simulink model "PV_solarpannel"  (R2019b)
settings: Solver=ode45  StartTime=0.0  StopTime=10.0  RelTol=1e-3  EnableMultiTasking=on
libraries: ee_lib x243, fl_lib x39, nesl_utility x11
(part 2 of 4)

== system PV_solarpannel/Subsystem1/Subsystem9/Subsystem4 ==
  Solar Cell : ee_lib/Sources/Solar Cell  prm=1  Isc=6 A  Voc=0.6 V  Is=1e-6 A  Is2=0 A  Iph=7.34 A  Ir0=1000 W/m^2  ec=1.5  N2=2  Rs=0 Ohm  Rp=Inf Ohm  N_series=1  TIPH1=0 1/K  EG=1.11 eV  TXIS1=3  TXIS2=3  TRS1=0  TRP1=0  Tmeas=25 C  TFIXED=25 C  thermal_mass=100 J/K  initial_temperature=25 degC
      settings: SourceProductName=Simscape Electrical  SourceProductBaseCode=PS
  Solar Cell1 : ee_lib/Sources/Solar Cell  prm=1  Isc=6 A  Voc=0.6 V  Is=1e-6 A  Is2=0 A  Iph=7.34 A  Ir0=1000 W/m^2  ec=1.5  N2=2  Rs=0 Ohm  Rp=Inf Ohm  N_series=1  TIPH1=0 1/K  EG=1.11 eV  TXIS1=3  TXIS2=3  TRS1=0  TRP1=0  Tmeas=25 C  TFIXED=25 C  thermal_mass=100 J/K  initial_temperature=25 degC
      settings: SourceProductName=Simscape Electrical  SourceProductBaseCode=PS
  Solar Cell2 : ee_lib/Sources/Solar Cell  prm=1  Isc=6 A  Voc=0.6 V  Is=1e-6 A  Is2=0 A  Iph=7.34 A  Ir0=1000 W/m^2  ec=1.5  N2=2  Rs=0 Ohm  Rp=Inf Ohm  N_series=1  TIPH1=0 1/K  EG=1.11 eV  TXIS1=3  TXIS2=3  TRS1=0  TRP1=0  Tmeas=25 C  TFIXED=25 C  thermal_mass=100 J/K  initial_temperature=25 degC
      settings: SourceProductName=Simscape Electrical  SourceProductBaseCode=PS
  Conn1 : PMIOPort  Side=Left
  Conn2 : PMIOPort  Port=2  Side=Right
  Conn3 : PMIOPort  Port=3  Side=Left
  connections:
  Solar Cell/LConn2 -- Conn2/RConn1
  Solar Cell/LConn1 -- Conn1/RConn1 -- Solar Cell2/LConn1 -- Solar Cell1/LConn1
  Solar Cell1/RConn1 -- Solar Cell2/LConn2
  Solar Cell/RConn1 -- Solar Cell1/LConn2
  Solar Cell2/RConn1 -- Conn3/RConn1

== system PV_solarpannel/Subsystem1/Subsystem9/Subsystem5 ==
  Solar Cell : ee_lib/Sources/Solar Cell  prm=1  Isc=6 A  Voc=0.6 V  Is=1e-6 A  Is2=0 A  Iph=7.34 A  Ir0=1000 W/m^2  ec=1.5  N2=2  Rs=0 Ohm  Rp=Inf Ohm  N_series=1  TIPH1=0 1/K  EG=1.11 eV  TXIS1=3  TXIS2=3  TRS1=0  TRP1=0  Tmeas=25 C  TFIXED=25 C  thermal_mass=100 J/K  initial_temperature=25 degC
      settings: SourceProductName=Simscape Electrical  SourceProductBaseCode=PS
  Solar Cell1 : ee_lib/Sources/Solar Cell  prm=1  Isc=6 A  Voc=0.6 V  Is=1e-6 A  Is2=0 A  Iph=7.34 A  Ir0=1000 W/m^2  ec=1.5  N2=2  Rs=0 Ohm  Rp=Inf Ohm  N_series=1  TIPH1=0 1/K  EG=1.11 eV  TXIS1=3  TXIS2=3  TRS1=0  TRP1=0  Tmeas=25 C  TFIXED=25 C  thermal_mass=100 J/K  initial_temperature=25 degC
      settings: SourceProductName=Simscape Electrical  SourceProductBaseCode=PS
  Solar Cell2 : ee_lib/Sources/Solar Cell  prm=1  Isc=6 A  Voc=0.6 V  Is=1e-6 A  Is2=0 A  Iph=7.34 A  Ir0=1000 W/m^2  ec=1.5  N2=2  Rs=0 Ohm  Rp=Inf Ohm  N_series=1  TIPH1=0 1/K  EG=1.11 eV  TXIS1=3  TXIS2=3  TRS1=0  TRP1=0  Tmeas=25 C  TFIXED=25 C  thermal_mass=100 J/K  initial_temperature=25 degC
      settings: SourceProductName=Simscape Electrical  SourceProductBaseCode=PS
  Conn1 : PMIOPort  Side=Left
  Conn2 : PMIOPort  Port=2  Side=Right
  Conn3 : PMIOPort  Port=3  Side=Left
  connections:
  Solar Cell/LConn2 -- Conn2/RConn1
  Solar Cell/LConn1 -- Conn1/RConn1 -- Solar Cell2/LConn1 -- Solar Cell1/LConn1
  Solar Cell1/RConn1 -- Solar Cell2/LConn2
  Solar Cell/RConn1 -- Solar Cell1/LConn2
  Solar Cell2/RConn1 -- Conn3/RConn1

== system PV_solarpannel/Subsystem1/Subsystem9/Subsystem6 ==
  Solar Cell : ee_lib/Sources/Solar Cell  prm=1  Isc=6 A  Voc=0.6 V  Is=1e-6 A  Is2=0 A  Iph=7.34 A  Ir0=1000 W/m^2  ec=1.5  N2=2  Rs=0 Ohm  Rp=Inf Ohm  N_series=1  TIPH1=0 1/K  EG=1.11 eV  TXIS1=3  TXIS2=3  TRS1=0  TRP1=0  Tmeas=25 C  TFIXED=25 C  thermal_mass=100 J/K  initial_temperature=25 degC
      settings: SourceProductName=Simscape Electrical  SourceProductBaseCode=PS
  Solar Cell1 : ee_lib/Sources/Solar Cell  prm=1  Isc=6 A  Voc=0.6 V  Is=1e-6 A  Is2=0 A  Iph=7.34 A  Ir0=1000 W/m^2  ec=1.5  N2=2  Rs=0 Ohm  Rp=Inf Ohm  N_series=1  TIPH1=0 1/K  EG=1.11 eV  TXIS1=3  TXIS2=3  TRS1=0  TRP1=0  Tmeas=25 C  TFIXED=25 C  thermal_mass=100 J/K  initial_temperature=25 degC
      settings: SourceProductName=Simscape Electrical  SourceProductBaseCode=PS
  Solar Cell2 : ee_lib/Sources/Solar Cell  prm=1  Isc=6 A  Voc=0.6 V  Is=1e-6 A  Is2=0 A  Iph=7.34 A  Ir0=1000 W/m^2  ec=1.5  N2=2  Rs=0 Ohm  Rp=Inf Ohm  N_series=1  TIPH1=0 1/K  EG=1.11 eV  TXIS1=3  TXIS2=3  TRS1=0  TRP1=0  Tmeas=25 C  TFIXED=25 C  thermal_mass=100 J/K  initial_temperature=25 degC
      settings: SourceProductName=Simscape Electrical  SourceProductBaseCode=PS
  Conn1 : PMIOPort  Side=Left
  Conn2 : PMIOPort  Port=2  Side=Right
  Conn3 : PMIOPort  Port=3  Side=Left
  connections:
  Solar Cell/LConn2 -- Conn2/RConn1
  Solar Cell/LConn1 -- Conn1/RConn1 -- Solar Cell2/LConn1 -- Solar Cell1/LConn1
  Solar Cell1/RConn1 -- Solar Cell2/LConn2
  Solar Cell/RConn1 -- Solar Cell1/LConn2
  Solar Cell2/RConn1 -- Conn3/RConn1

== system PV_solarpannel/Subsystem1/Subsystem9/Subsystem7 ==
  Solar Cell : ee_lib/Sources/Solar Cell  prm=1  Isc=6 A  Voc=0.6 V  Is=1e-6 A  Is2=0 A  Iph=7.34 A  Ir0=1000 W/m^2  ec=1.5  N2=2  Rs=0 Ohm  Rp=Inf Ohm  N_series=1  TIPH1=0 1/K  EG=1.11 eV  TXIS1=3  TXIS2=3  TRS1=0  TRP1=0  Tmeas=25 C  TFIXED=25 C  thermal_mass=100 J/K  initial_temperature=25 degC
      settings: SourceProductName=Simscape Electrical  SourceProductBaseCode=PS
  Solar Cell1 : ee_lib/Sources/Solar Cell  prm=1  Isc=6 A  Voc=0.6 V  Is=1e-6 A  Is2=0 A  Iph=7.34 A  Ir0=1000 W/m^2  ec=1.5  N2=2  Rs=0 Ohm  Rp=Inf Ohm  N_series=1  TIPH1=0 1/K  EG=1.11 eV  TXIS1=3  TXIS2=3  TRS1=0  TRP1=0  Tmeas=25 C  TFIXED=25 C  thermal_mass=100 J/K  initial_temperature=25 degC
      settings: SourceProductName=Simscape Electrical  SourceProductBaseCode=PS
  Solar Cell2 : ee_lib/Sources/Solar Cell  prm=1  Isc=6 A  Voc=0.6 V  Is=1e-6 A  Is2=0 A  Iph=7.34 A  Ir0=1000 W/m^2  ec=1.5  N2=2  Rs=0 Ohm  Rp=Inf Ohm  N_series=1  TIPH1=0 1/K  EG=1.11 eV  TXIS1=3  TXIS2=3  TRS1=0  TRP1=0  Tmeas=25 C  TFIXED=25 C  thermal_mass=100 J/K  initial_temperature=25 degC
      settings: SourceProductName=Simscape Electrical  SourceProductBaseCode=PS
  Conn1 : PMIOPort  Side=Left
  Conn2 : PMIOPort  Port=2  Side=Right
  Conn3 : PMIOPort  Port=3  Side=Left
  connections:
  Solar Cell/LConn2 -- Conn2/RConn1
  Solar Cell/LConn1 -- Conn1/RConn1 -- Solar Cell2/LConn1 -- Solar Cell1/LConn1
  Solar Cell1/RConn1 -- Solar Cell2/LConn2
  Solar Cell/RConn1 -- Solar Cell1/LConn2
  Solar Cell2/RConn1 -- Conn3/RConn1

== system PV_solarpannel/Subsystem1/Subsystem9/Subsystem8 ==
  Solar Cell : ee_lib/Sources/Solar Cell  prm=1  Isc=6 A  Voc=0.6 V  Is=1e-6 A  Is2=0 A  Iph=7.34 A  Ir0=1000 W/m^2  ec=1.5  N2=2  Rs=0 Ohm  Rp=Inf Ohm  N_series=1  TIPH1=0 1/K  EG=1.11 eV  TXIS1=3  TXIS2=3  TRS1=0  TRP1=0  Tmeas=25 C  TFIXED=25 C  thermal_mass=100 J/K  initial_temperature=25 degC
      settings: SourceProductName=Simscape Electrical  SourceProductBaseCode=PS
  Solar Cell1 : ee_lib/Sources/Solar Cell  prm=1  Isc=6 A  Voc=0.6 V  Is=1e-6 A  Is2=0 A  Iph=7.34 A  Ir0=1000 W/m^2  ec=1.5  N2=2  Rs=0 Ohm  Rp=Inf Ohm  N_series=1  TIPH1=0 1/K  EG=1.11 eV  TXIS1=3  TXIS2=3  TRS1=0  TRP1=0  Tmeas=25 C  TFIXED=25 C  thermal_mass=100 J/K  initial_temperature=25 degC
      settings: SourceProductName=Simscape Electrical  SourceProductBaseCode=PS
  Solar Cell2 : ee_lib/Sources/Solar Cell  prm=1  Isc=6 A  Voc=0.6 V  Is=1e-6 A  Is2=0 A  Iph=7.34 A  Ir0=1000 W/m^2  ec=1.5  N2=2  Rs=0 Ohm  Rp=Inf Ohm  N_series=1  TIPH1=0 1/K  EG=1.11 eV  TXIS1=3  TXIS2=3  TRS1=0  TRP1=0  Tmeas=25 C  TFIXED=25 C  thermal_mass=100 J/K  initial_temperature=25 degC
      settings: SourceProductName=Simscape Electrical  SourceProductBaseCode=PS
  Conn1 : PMIOPort  Side=Left
  Conn2 : PMIOPort  Port=2  Side=Right
  Conn3 : PMIOPort  Port=3  Side=Left
  connections:
  Solar Cell/LConn2 -- Conn2/RConn1
  Solar Cell/LConn1 -- Conn1/RConn1 -- Solar Cell2/LConn1 -- Solar Cell1/LConn1
  Solar Cell1/RConn1 -- Solar Cell2/LConn2
  Solar Cell/RConn1 -- Solar Cell1/LConn2
  Solar Cell2/RConn1 -- Conn3/RConn1

== system PV_solarpannel/Subsystem2/Subsystem9/Subsystem ==
  Solar Cell : ee_lib/Sources/Solar Cell  prm=1  Isc=6 A  Voc=0.6 V  Is=1e-6 A  Is2=0 A  Iph=7.34 A  Ir0=1000 W/m^2  ec=1.5  N2=2  Rs=0 Ohm  Rp=Inf Ohm  N_series=1  TIPH1=0 1/K  EG=1.11 eV  TXIS1=3  TXIS2=3  TRS1=0  TRP1=0  Tmeas=25 C  TFIXED=25 C  thermal_mass=100 J/K  initial_temperature=25 degC
      settings: SourceProductName=Simscape Electrical  SourceProductBaseCode=PS
  Solar Cell1 : ee_lib/Sources/Solar Cell  prm=1  Isc=6 A  Voc=0.6 V  Is=1e-6 A  Is2=0 A  Iph=7.34 A  Ir0=1000 W/m^2  ec=1.5  N2=2  Rs=0 Ohm  Rp=Inf Ohm  N_series=1  TIPH1=0 1/K  EG=1.11 eV  TXIS1=3  TXIS2=3  TRS1=0  TRP1=0  Tmeas=25 C  TFIXED=25 C  thermal_mass=100 J/K  initial_temperature=25 degC
      settings: SourceProductName=Simscape Electrical  SourceProductBaseCode=PS
  Solar Cell2 : ee_lib/Sources/Solar Cell  prm=1  Isc=6 A  Voc=0.6 V  Is=1e-6 A  Is2=0 A  Iph=7.34 A  Ir0=1000 W/m^2  ec=1.5  N2=2  Rs=0 Ohm  Rp=Inf Ohm  N_series=1  TIPH1=0 1/K  EG=1.11 eV  TXIS1=3  TXIS2=3  TRS1=0  TRP1=0  Tmeas=25 C  TFIXED=25 C  thermal_mass=100 J/K  initial_temperature=25 degC
      settings: SourceProductName=Simscape Electrical  SourceProductBaseCode=PS
  Conn1 : PMIOPort  Side=Left
  Conn2 : PMIOPort  Port=2  Side=Right
  Conn3 : PMIOPort  Port=3  Side=Left
  connections:
  Solar Cell/LConn2 -- Conn2/RConn1
  Solar Cell/LConn1 -- Conn1/RConn1 -- Solar Cell2/LConn1 -- Solar Cell1/LConn1
  Solar Cell1/RConn1 -- Solar Cell2/LConn2
  Solar Cell/RConn1 -- Solar Cell1/LConn2
  Solar Cell2/RConn1 -- Conn3/RConn1

== system PV_solarpannel/Subsystem2/Subsystem9/Subsystem1 ==
  Solar Cell : ee_lib/Sources/Solar Cell  prm=1  Isc=6 A  Voc=0.6 V  Is=1e-6 A  Is2=0 A  Iph=7.34 A  Ir0=1000 W/m^2  ec=1.5  N2=2  Rs=0 Ohm  Rp=Inf Ohm  N_series=1  TIPH1=0 1/K  EG=1.11 eV  TXIS1=3  TXIS2=3  TRS1=0  TRP1=0  Tmeas=25 C  TFIXED=25 C  thermal_mass=100 J/K  initial_temperature=25 degC
      settings: SourceProductName=Simscape Electrical  SourceProductBaseCode=PS
  Solar Cell1 : ee_lib/Sources/Solar Cell  prm=1  Isc=6 A  Voc=0.6 V  Is=1e-6 A  Is2=0 A  Iph=7.34 A  Ir0=1000 W/m^2  ec=1.5  N2=2  Rs=0 Ohm  Rp=Inf Ohm  N_series=1  TIPH1=0 1/K  EG=1.11 eV  TXIS1=3  TXIS2=3  TRS1=0  TRP1=0  Tmeas=25 C  TFIXED=25 C  thermal_mass=100 J/K  initial_temperature=25 degC
      settings: SourceProductName=Simscape Electrical  SourceProductBaseCode=PS
  Solar Cell2 : ee_lib/Sources/Solar Cell  prm=1  Isc=6 A  Voc=0.6 V  Is=1e-6 A  Is2=0 A  Iph=7.34 A  Ir0=1000 W/m^2  ec=1.5  N2=2  Rs=0 Ohm  Rp=Inf Ohm  N_series=1  TIPH1=0 1/K  EG=1.11 eV  TXIS1=3  TXIS2=3  TRS1=0  TRP1=0  Tmeas=25 C  TFIXED=25 C  thermal_mass=100 J/K  initial_temperature=25 degC
      settings: SourceProductName=Simscape Electrical  SourceProductBaseCode=PS
  Conn1 : PMIOPort  Side=Left
  Conn2 : PMIOPort  Port=2  Side=Right
  Conn3 : PMIOPort  Port=3  Side=Left
  connections:
  Solar Cell2/RConn1 -- Conn3/RConn1
  Solar Cell/RConn1 -- Solar Cell1/LConn2
  Solar Cell1/RConn1 -- Solar Cell2/LConn2
  Conn1/RConn1 -- Solar Cell/LConn1 -- Solar Cell1/LConn1 -- Solar Cell2/LConn1
  Solar Cell/LConn2 -- Conn2/RConn1

== system PV_solarpannel/Subsystem2/Subsystem9/Subsystem2 ==
  Solar Cell : ee_lib/Sources/Solar Cell  prm=1  Isc=6 A  Voc=0.6 V  Is=1e-6 A  Is2=0 A  Iph=7.34 A  Ir0=1000 W/m^2  ec=1.5  N2=2  Rs=0 Ohm  Rp=Inf Ohm  N_series=1  TIPH1=0 1/K  EG=1.11 eV  TXIS1=3  TXIS2=3  TRS1=0  TRP1=0  Tmeas=25 C  TFIXED=25 C  thermal_mass=100 J/K  initial_temperature=25 degC
      settings: SourceProductName=Simscape Electrical  SourceProductBaseCode=PS
  Solar Cell1 : ee_lib/Sources/Solar Cell  prm=1  Isc=6 A  Voc=0.6 V  Is=1e-6 A  Is2=0 A  Iph=7.34 A  Ir0=1000 W/m^2  ec=1.5  N2=2  Rs=0 Ohm  Rp=Inf Ohm  N_series=1  TIPH1=0 1/K  EG=1.11 eV  TXIS1=3  TXIS2=3  TRS1=0  TRP1=0  Tmeas=25 C  TFIXED=25 C  thermal_mass=100 J/K  initial_temperature=25 degC
      settings: SourceProductName=Simscape Electrical  SourceProductBaseCode=PS
  Solar Cell2 : ee_lib/Sources/Solar Cell  prm=1  Isc=6 A  Voc=0.6 V  Is=1e-6 A  Is2=0 A  Iph=7.34 A  Ir0=1000 W/m^2  ec=1.5  N2=2  Rs=0 Ohm  Rp=Inf Ohm  N_series=1  TIPH1=0 1/K  EG=1.11 eV  TXIS1=3  TXIS2=3  TRS1=0  TRP1=0  Tmeas=25 C  TFIXED=25 C  thermal_mass=100 J/K  initial_temperature=25 degC
      settings: SourceProductName=Simscape Electrical  SourceProductBaseCode=PS
  Conn1 : PMIOPort  Side=Left
  Conn2 : PMIOPort  Port=2  Side=Right
  Conn3 : PMIOPort  Port=3  Side=Left
  connections:
  Solar Cell/LConn2 -- Conn2/RConn1
  Solar Cell2/LConn1 -- Solar Cell1/LConn1 -- Solar Cell/LConn1 -- Conn1/RConn1
  Solar Cell1/RConn1 -- Solar Cell2/LConn2
  Solar Cell/RConn1 -- Solar Cell1/LConn2
  Solar Cell2/RConn1 -- Conn3/RConn1

== system PV_solarpannel/Subsystem2/Subsystem9/Subsystem3 ==
  Solar Cell : ee_lib/Sources/Solar Cell  prm=1  Isc=6 A  Voc=0.6 V  Is=1e-6 A  Is2=0 A  Iph=7.34 A  Ir0=1000 W/m^2  ec=1.5  N2=2  Rs=0 Ohm  Rp=Inf Ohm  N_series=1  TIPH1=0 1/K  EG=1.11 eV  TXIS1=3  TXIS2=3  TRS1=0  TRP1=0  Tmeas=25 C  TFIXED=25 C  thermal_mass=100 J/K  initial_temperature=25 degC
      settings: SourceProductName=Simscape Electrical  SourceProductBaseCode=PS
  Solar Cell1 : ee_lib/Sources/Solar Cell  prm=1  Isc=6 A  Voc=0.6 V  Is=1e-6 A  Is2=0 A  Iph=7.34 A  Ir0=1000 W/m^2  ec=1.5  N2=2  Rs=0 Ohm  Rp=Inf Ohm  N_series=1  TIPH1=0 1/K  EG=1.11 eV  TXIS1=3  TXIS2=3  TRS1=0  TRP1=0  Tmeas=25 C  TFIXED=25 C  thermal_mass=100 J/K  initial_temperature=25 degC
      settings: SourceProductName=Simscape Electrical  SourceProductBaseCode=PS
  Solar Cell2 : ee_lib/Sources/Solar Cell  prm=1  Isc=6 A  Voc=0.6 V  Is=1e-6 A  Is2=0 A  Iph=7.34 A  Ir0=1000 W/m^2  ec=1.5  N2=2  Rs=0 Ohm  Rp=Inf Ohm  N_series=1  TIPH1=0 1/K  EG=1.11 eV  TXIS1=3  TXIS2=3  TRS1=0  TRP1=0  Tmeas=25 C  TFIXED=25 C  thermal_mass=100 J/K  initial_temperature=25 degC
      settings: SourceProductName=Simscape Electrical  SourceProductBaseCode=PS
  Conn1 : PMIOPort  Side=Left
  Conn2 : PMIOPort  Port=2  Side=Right
  Conn3 : PMIOPort  Port=3  Side=Left
  connections:
  Solar Cell/LConn2 -- Conn2/RConn1
  Solar Cell/LConn1 -- Conn1/RConn1 -- Solar Cell2/LConn1 -- Solar Cell1/LConn1
  Solar Cell1/RConn1 -- Solar Cell2/LConn2
  Solar Cell/RConn1 -- Solar Cell1/LConn2
  Solar Cell2/RConn1 -- Conn3/RConn1

== system PV_solarpannel/Subsystem2/Subsystem9/Subsystem4 ==
  Solar Cell : ee_lib/Sources/Solar Cell  prm=1  Isc=6 A  Voc=0.6 V  Is=1e-6 A  Is2=0 A  Iph=7.34 A  Ir0=1000 W/m^2  ec=1.5  N2=2  Rs=0 Ohm  Rp=Inf Ohm  N_series=1  TIPH1=0 1/K  EG=1.11 eV  TXIS1=3  TXIS2=3  TRS1=0  TRP1=0  Tmeas=25 C  TFIXED=25 C  thermal_mass=100 J/K  initial_temperature=25 degC
      settings: SourceProductName=Simscape Electrical  SourceProductBaseCode=PS
  Solar Cell1 : ee_lib/Sources/Solar Cell  prm=1  Isc=6 A  Voc=0.6 V  Is=1e-6 A  Is2=0 A  Iph=7.34 A  Ir0=1000 W/m^2  ec=1.5  N2=2  Rs=0 Ohm  Rp=Inf Ohm  N_series=1  TIPH1=0 1/K  EG=1.11 eV  TXIS1=3  TXIS2=3  TRS1=0  TRP1=0  Tmeas=25 C  TFIXED=25 C  thermal_mass=100 J/K  initial_temperature=25 degC
      settings: SourceProductName=Simscape Electrical  SourceProductBaseCode=PS
  Solar Cell2 : ee_lib/Sources/Solar Cell  prm=1  Isc=6 A  Voc=0.6 V  Is=1e-6 A  Is2=0 A  Iph=7.34 A  Ir0=1000 W/m^2  ec=1.5  N2=2  Rs=0 Ohm  Rp=Inf Ohm  N_series=1  TIPH1=0 1/K  EG=1.11 eV  TXIS1=3  TXIS2=3  TRS1=0  TRP1=0  Tmeas=25 C  TFIXED=25 C  thermal_mass=100 J/K  initial_temperature=25 degC
      settings: SourceProductName=Simscape Electrical  SourceProductBaseCode=PS
  Conn1 : PMIOPort  Side=Left
  Conn2 : PMIOPort  Port=2  Side=Right
  Conn3 : PMIOPort  Port=3  Side=Left
  connections:
  Solar Cell/LConn2 -- Conn2/RConn1
  Solar Cell/LConn1 -- Conn1/RConn1 -- Solar Cell2/LConn1 -- Solar Cell1/LConn1
  Solar Cell1/RConn1 -- Solar Cell2/LConn2
  Solar Cell/RConn1 -- Solar Cell1/LConn2
  Solar Cell2/RConn1 -- Conn3/RConn1

== system PV_solarpannel/Subsystem2/Subsystem9/Subsystem5 ==
  Solar Cell : ee_lib/Sources/Solar Cell  prm=1  Isc=6 A  Voc=0.6 V  Is=1e-6 A  Is2=0 A  Iph=7.34 A  Ir0=1000 W/m^2  ec=1.5  N2=2  Rs=0 Ohm  Rp=Inf Ohm  N_series=1  TIPH1=0 1/K  EG=1.11 eV  TXIS1=3  TXIS2=3  TRS1=0  TRP1=0  Tmeas=25 C  TFIXED=25 C  thermal_mass=100 J/K  initial_temperature=25 degC
      settings: SourceProductName=Simscape Electrical  SourceProductBaseCode=PS
  Solar Cell1 : ee_lib/Sources/Solar Cell  prm=1  Isc=6 A  Voc=0.6 V  Is=1e-6 A  Is2=0 A  Iph=7.34 A  Ir0=1000 W/m^2  ec=1.5  N2=2  Rs=0 Ohm  Rp=Inf Ohm  N_series=1  TIPH1=0 1/K  EG=1.11 eV  TXIS1=3  TXIS2=3  TRS1=0  TRP1=0  Tmeas=25 C  TFIXED=25 C  thermal_mass=100 J/K  initial_temperature=25 degC
      settings: SourceProductName=Simscape Electrical  SourceProductBaseCode=PS
  Solar Cell2 : ee_lib/Sources/Solar Cell  prm=1  Isc=6 A  Voc=0.6 V  Is=1e-6 A  Is2=0 A  Iph=7.34 A  Ir0=1000 W/m^2  ec=1.5  N2=2  Rs=0 Ohm  Rp=Inf Ohm  N_series=1  TIPH1=0 1/K  EG=1.11 eV  TXIS1=3  TXIS2=3  TRS1=0  TRP1=0  Tmeas=25 C  TFIXED=25 C  thermal_mass=100 J/K  initial_temperature=25 degC
      settings: SourceProductName=Simscape Electrical  SourceProductBaseCode=PS
  Conn1 : PMIOPort  Side=Left
  Conn2 : PMIOPort  Port=2  Side=Right
  Conn3 : PMIOPort  Port=3  Side=Left
  connections:
  Solar Cell/LConn2 -- Conn2/RConn1
  Solar Cell/LConn1 -- Conn1/RConn1 -- Solar Cell2/LConn1 -- Solar Cell1/LConn1
  Solar Cell1/RConn1 -- Solar Cell2/LConn2
  Solar Cell/RConn1 -- Solar Cell1/LConn2
  Solar Cell2/RConn1 -- Conn3/RConn1

== system PV_solarpannel/Subsystem2/Subsystem9/Subsystem6 ==
  Solar Cell : ee_lib/Sources/Solar Cell  prm=1  Isc=6 A  Voc=0.6 V  Is=1e-6 A  Is2=0 A  Iph=7.34 A  Ir0=1000 W/m^2  ec=1.5  N2=2  Rs=0 Ohm  Rp=Inf Ohm  N_series=1  TIPH1=0 1/K  EG=1.11 eV  TXIS1=3  TXIS2=3  TRS1=0  TRP1=0  Tmeas=25 C  TFIXED=25 C  thermal_mass=100 J/K  initial_temperature=25 degC
      settings: SourceProductName=Simscape Electrical  SourceProductBaseCode=PS
  Solar Cell1 : ee_lib/Sources/Solar Cell  prm=1  Isc=6 A  Voc=0.6 V  Is=1e-6 A  Is2=0 A  Iph=7.34 A  Ir0=1000 W/m^2  ec=1.5  N2=2  Rs=0 Ohm  Rp=Inf Ohm  N_series=1  TIPH1=0 1/K  EG=1.11 eV  TXIS1=3  TXIS2=3  TRS1=0  TRP1=0  Tmeas=25 C  TFIXED=25 C  thermal_mass=100 J/K  initial_temperature=25 degC
      settings: SourceProductName=Simscape Electrical  SourceProductBaseCode=PS
  Solar Cell2 : ee_lib/Sources/Solar Cell  prm=1  Isc=6 A  Voc=0.6 V  Is=1e-6 A  Is2=0 A  Iph=7.34 A  Ir0=1000 W/m^2  ec=1.5  N2=2  Rs=0 Ohm  Rp=Inf Ohm  N_series=1  TIPH1=0 1/K  EG=1.11 eV  TXIS1=3  TXIS2=3  TRS1=0  TRP1=0  Tmeas=25 C  TFIXED=25 C  thermal_mass=100 J/K  initial_temperature=25 degC
      settings: SourceProductName=Simscape Electrical  SourceProductBaseCode=PS
  Conn1 : PMIOPort  Side=Left
  Conn2 : PMIOPort  Port=2  Side=Right
  Conn3 : PMIOPort  Port=3  Side=Left
  connections:
  Solar Cell/LConn2 -- Conn2/RConn1
  Solar Cell/LConn1 -- Conn1/RConn1 -- Solar Cell2/LConn1 -- Solar Cell1/LConn1
  Solar Cell1/RConn1 -- Solar Cell2/LConn2
  Solar Cell/RConn1 -- Solar Cell1/LConn2
  Solar Cell2/RConn1 -- Conn3/RConn1

== system PV_solarpannel/Subsystem2/Subsystem9/Subsystem7 ==
  Solar Cell : ee_lib/Sources/Solar Cell  prm=1  Isc=6 A  Voc=0.6 V  Is=1e-6 A  Is2=0 A  Iph=7.34 A  Ir0=1000 W/m^2  ec=1.5  N2=2  Rs=0 Ohm  Rp=Inf Ohm  N_series=1  TIPH1=0 1/K  EG=1.11 eV  TXIS1=3  TXIS2=3  TRS1=0  TRP1=0  Tmeas=25 C  TFIXED=25 C  thermal_mass=100 J/K  initial_temperature=25 degC
      settings: SourceProductName=Simscape Electrical  SourceProductBaseCode=PS
  Solar Cell1 : ee_lib/Sources/Solar Cell  prm=1  Isc=6 A  Voc=0.6 V  Is=1e-6 A  Is2=0 A  Iph=7.34 A  Ir0=1000 W/m^2  ec=1.5  N2=2  Rs=0 Ohm  Rp=Inf Ohm  N_series=1  TIPH1=0 1/K  EG=1.11 eV  TXIS1=3  TXIS2=3  TRS1=0  TRP1=0  Tmeas=25 C  TFIXED=25 C  thermal_mass=100 J/K  initial_temperature=25 degC
      settings: SourceProductName=Simscape Electrical  SourceProductBaseCode=PS
  Solar Cell2 : ee_lib/Sources/Solar Cell  prm=1  Isc=6 A  Voc=0.6 V  Is=1e-6 A  Is2=0 A  Iph=7.34 A  Ir0=1000 W/m^2  ec=1.5  N2=2  Rs=0 Ohm  Rp=Inf Ohm  N_series=1  TIPH1=0 1/K  EG=1.11 eV  TXIS1=3  TXIS2=3  TRS1=0  TRP1=0  Tmeas=25 C  TFIXED=25 C  thermal_mass=100 J/K  initial_temperature=25 degC
      settings: SourceProductName=Simscape Electrical  SourceProductBaseCode=PS
  Conn1 : PMIOPort  Side=Left
  Conn2 : PMIOPort  Port=2  Side=Right
  Conn3 : PMIOPort  Port=3  Side=Left
  connections:
  Solar Cell/LConn2 -- Conn2/RConn1
  Solar Cell/LConn1 -- Conn1/RConn1 -- Solar Cell2/LConn1 -- Solar Cell1/LConn1
  Solar Cell1/RConn1 -- Solar Cell2/LConn2
  Solar Cell/RConn1 -- Solar Cell1/LConn2
  Solar Cell2/RConn1 -- Conn3/RConn1

== system PV_solarpannel/Subsystem2/Subsystem9/Subsystem8 ==
  Solar Cell : ee_lib/Sources/Solar Cell  prm=1  Isc=6 A  Voc=0.6 V  Is=1e-6 A  Is2=0 A  Iph=7.34 A  Ir0=1000 W/m^2  ec=1.5  N2=2  Rs=0 Ohm  Rp=Inf Ohm  N_series=1  TIPH1=0 1/K  EG=1.11 eV  TXIS1=3  TXIS2=3  TRS1=0  TRP1=0  Tmeas=25 C  TFIXED=25 C  thermal_mass=100 J/K  initial_temperature=25 degC
      settings: SourceProductName=Simscape Electrical  SourceProductBaseCode=PS
  Solar Cell1 : ee_lib/Sources/Solar Cell  prm=1  Isc=6 A  Voc=0.6 V  Is=1e-6 A  Is2=0 A  Iph=7.34 A  Ir0=1000 W/m^2  ec=1.5  N2=2  Rs=0 Ohm  Rp=Inf Ohm  N_series=1  TIPH1=0 1/K  EG=1.11 eV  TXIS1=3  TXIS2=3  TRS1=0  TRP1=0  Tmeas=25 C  TFIXED=25 C  thermal_mass=100 J/K  initial_temperature=25 degC
      settings: SourceProductName=Simscape Electrical  SourceProductBaseCode=PS
  Solar Cell2 : ee_lib/Sources/Solar Cell  prm=1  Isc=6 A  Voc=0.6 V  Is=1e-6 A  Is2=0 A  Iph=7.34 A  Ir0=1000 W/m^2  ec=1.5  N2=2  Rs=0 Ohm  Rp=Inf Ohm  N_series=1  TIPH1=0 1/K  EG=1.11 eV  TXIS1=3  TXIS2=3  TRS1=0  TRP1=0  Tmeas=25 C  TFIXED=25 C  thermal_mass=100 J/K  initial_temperature=25 degC
      settings: SourceProductName=Simscape Electrical  SourceProductBaseCode=PS
  Conn1 : PMIOPort  Side=Left
  Conn2 : PMIOPort  Port=2  Side=Right
  Conn3 : PMIOPort  Port=3  Side=Left
  connections:
  Solar Cell/LConn2 -- Conn2/RConn1
  Solar Cell/LConn1 -- Conn1/RConn1 -- Solar Cell2/LConn1 -- Solar Cell1/LConn1
  Solar Cell1/RConn1 -- Solar Cell2/LConn2
  Solar Cell/RConn1 -- Solar Cell1/LConn2
  Solar Cell2/RConn1 -- Conn3/RConn1

== system PV_solarpannel/Subsystem3/Subsystem9/Subsystem ==
  Solar Cell : ee_lib/Sources/Solar Cell  prm=1  Isc=6 A  Voc=0.6 V  Is=1e-6 A  Is2=0 A  Iph=7.34 A  Ir0=1000 W/m^2  ec=1.5  N2=2  Rs=0 Ohm  Rp=Inf Ohm  N_series=1  TIPH1=0 1/K  EG=1.11 eV  TXIS1=3  TXIS2=3  TRS1=0  TRP1=0  Tmeas=25 C  TFIXED=25 C  thermal_mass=100 J/K  initial_temperature=25 degC
      settings: SourceProductName=Simscape Electrical  SourceProductBaseCode=PS
  Solar Cell1 : ee_lib/Sources/Solar Cell  prm=1  Isc=6 A  Voc=0.6 V  Is=1e-6 A  Is2=0 A  Iph=7.34 A  Ir0=1000 W/m^2  ec=1.5  N2=2  Rs=0 Ohm  Rp=Inf Ohm  N_series=1  TIPH1=0 1/K  EG=1.11 eV  TXIS1=3  TXIS2=3  TRS1=0  TRP1=0  Tmeas=25 C  TFIXED=25 C  thermal_mass=100 J/K  initial_temperature=25 degC
      settings: SourceProductName=Simscape Electrical  SourceProductBaseCode=PS
  Solar Cell2 : ee_lib/Sources/Solar Cell  prm=1  Isc=6 A  Voc=0.6 V  Is=1e-6 A  Is2=0 A  Iph=7.34 A  Ir0=1000 W/m^2  ec=1.5  N2=2  Rs=0 Ohm  Rp=Inf Ohm  N_series=1  TIPH1=0 1/K  EG=1.11 eV  TXIS1=3  TXIS2=3  TRS1=0  TRP1=0  Tmeas=25 C  TFIXED=25 C  thermal_mass=100 J/K  initial_temperature=25 degC
      settings: SourceProductName=Simscape Electrical  SourceProductBaseCode=PS
  Conn1 : PMIOPort  Side=Left
  Conn2 : PMIOPort  Port=2  Side=Right
  Conn3 : PMIOPort  Port=3  Side=Left
  connections:
  Solar Cell/LConn2 -- Conn2/RConn1
  Solar Cell/LConn1 -- Conn1/RConn1 -- Solar Cell2/LConn1 -- Solar Cell1/LConn1
  Solar Cell1/RConn1 -- Solar Cell2/LConn2
  Solar Cell/RConn1 -- Solar Cell1/LConn2
  Solar Cell2/RConn1 -- Conn3/RConn1

== system PV_solarpannel/Subsystem3/Subsystem9/Subsystem1 ==
  Solar Cell : ee_lib/Sources/Solar Cell  prm=1  Isc=6 A  Voc=0.6 V  Is=1e-6 A  Is2=0 A  Iph=7.34 A  Ir0=1000 W/m^2  ec=1.5  N2=2  Rs=0 Ohm  Rp=Inf Ohm  N_series=1  TIPH1=0 1/K  EG=1.11 eV  TXIS1=3  TXIS2=3  TRS1=0  TRP1=0  Tmeas=25 C  TFIXED=25 C  thermal_mass=100 J/K  initial_temperature=25 degC
      settings: SourceProductName=Simscape Electrical  SourceProductBaseCode=PS
  Solar Cell1 : ee_lib/Sources/Solar Cell  prm=1  Isc=6 A  Voc=0.6 V  Is=1e-6 A  Is2=0 A  Iph=7.34 A  Ir0=1000 W/m^2  ec=1.5  N2=2  Rs=0 Ohm  Rp=Inf Ohm  N_series=1  TIPH1=0 1/K  EG=1.11 eV  TXIS1=3  TXIS2=3  TRS1=0  TRP1=0  Tmeas=25 C  TFIXED=25 C  thermal_mass=100 J/K  initial_temperature=25 degC
      settings: SourceProductName=Simscape Electrical  SourceProductBaseCode=PS
  Solar Cell2 : ee_lib/Sources/Solar Cell  prm=1  Isc=6 A  Voc=0.6 V  Is=1e-6 A  Is2=0 A  Iph=7.34 A  Ir0=1000 W/m^2  ec=1.5  N2=2  Rs=0 Ohm  Rp=Inf Ohm  N_series=1  TIPH1=0 1/K  EG=1.11 eV  TXIS1=3  TXIS2=3  TRS1=0  TRP1=0  Tmeas=25 C  TFIXED=25 C  thermal_mass=100 J/K  initial_temperature=25 degC
      settings: SourceProductName=Simscape Electrical  SourceProductBaseCode=PS
  Conn1 : PMIOPort  Side=Left
  Conn2 : PMIOPort  Port=2  Side=Right
  Conn3 : PMIOPort  Port=3  Side=Left
  connections:
  Solar Cell2/RConn1 -- Conn3/RConn1
  Solar Cell/RConn1 -- Solar Cell1/LConn2
  Solar Cell1/RConn1 -- Solar Cell2/LConn2
  Conn1/RConn1 -- Solar Cell/LConn1 -- Solar Cell1/LConn1 -- Solar Cell2/LConn1
  Solar Cell/LConn2 -- Conn2/RConn1

== system PV_solarpannel/Subsystem3/Subsystem9/Subsystem2 ==
  Solar Cell : ee_lib/Sources/Solar Cell  prm=1  Isc=6 A  Voc=0.6 V  Is=1e-6 A  Is2=0 A  Iph=7.34 A  Ir0=1000 W/m^2  ec=1.5  N2=2  Rs=0 Ohm  Rp=Inf Ohm  N_series=1  TIPH1=0 1/K  EG=1.11 eV  TXIS1=3  TXIS2=3  TRS1=0  TRP1=0  Tmeas=25 C  TFIXED=25 C  thermal_mass=100 J/K  initial_temperature=25 degC
      settings: SourceProductName=Simscape Electrical  SourceProductBaseCode=PS
  Solar Cell1 : ee_lib/Sources/Solar Cell  prm=1  Isc=6 A  Voc=0.6 V  Is=1e-6 A  Is2=0 A  Iph=7.34 A  Ir0=1000 W/m^2  ec=1.5  N2=2  Rs=0 Ohm  Rp=Inf Ohm  N_series=1  TIPH1=0 1/K  EG=1.11 eV  TXIS1=3  TXIS2=3  TRS1=0  TRP1=0  Tmeas=25 C  TFIXED=25 C  thermal_mass=100 J/K  initial_temperature=25 degC
      settings: SourceProductName=Simscape Electrical  SourceProductBaseCode=PS
  Solar Cell2 : ee_lib/Sources/Solar Cell  prm=1  Isc=6 A  Voc=0.6 V  Is=1e-6 A  Is2=0 A  Iph=7.34 A  Ir0=1000 W/m^2  ec=1.5  N2=2  Rs=0 Ohm  Rp=Inf Ohm  N_series=1  TIPH1=0 1/K  EG=1.11 eV  TXIS1=3  TXIS2=3  TRS1=0  TRP1=0  Tmeas=25 C  TFIXED=25 C  thermal_mass=100 J/K  initial_temperature=25 degC
      settings: SourceProductName=Simscape Electrical  SourceProductBaseCode=PS
  Conn1 : PMIOPort  Side=Left
  Conn2 : PMIOPort  Port=2  Side=Right
  Conn3 : PMIOPort  Port=3  Side=Left
  connections:
  Solar Cell/LConn2 -- Conn2/RConn1
  Solar Cell2/LConn1 -- Solar Cell1/LConn1 -- Solar Cell/LConn1 -- Conn1/RConn1
  Solar Cell1/RConn1 -- Solar Cell2/LConn2
  Solar Cell/RConn1 -- Solar Cell1/LConn2
  Solar Cell2/RConn1 -- Conn3/RConn1

== system PV_solarpannel/Subsystem3/Subsystem9/Subsystem3 ==
  Solar Cell : ee_lib/Sources/Solar Cell  prm=1  Isc=6 A  Voc=0.6 V  Is=1e-6 A  Is2=0 A  Iph=7.34 A  Ir0=1000 W/m^2  ec=1.5  N2=2  Rs=0 Ohm  Rp=Inf Ohm  N_series=1  TIPH1=0 1/K  EG=1.11 eV  TXIS1=3  TXIS2=3  TRS1=0  TRP1=0  Tmeas=25 C  TFIXED=25 C  thermal_mass=100 J/K  initial_temperature=25 degC
      settings: SourceProductName=Simscape Electrical  SourceProductBaseCode=PS
  Solar Cell1 : ee_lib/Sources/Solar Cell  prm=1  Isc=6 A  Voc=0.6 V  Is=1e-6 A  Is2=0 A  Iph=7.34 A  Ir0=1000 W/m^2  ec=1.5  N2=2  Rs=0 Ohm  Rp=Inf Ohm  N_series=1  TIPH1=0 1/K  EG=1.11 eV  TXIS1=3  TXIS2=3  TRS1=0  TRP1=0  Tmeas=25 C  TFIXED=25 C  thermal_mass=100 J/K  initial_temperature=25 degC
      settings: SourceProductName=Simscape Electrical  SourceProductBaseCode=PS
  Solar Cell2 : ee_lib/Sources/Solar Cell  prm=1  Isc=6 A  Voc=0.6 V  Is=1e-6 A  Is2=0 A  Iph=7.34 A  Ir0=1000 W/m^2  ec=1.5  N2=2  Rs=0 Ohm  Rp=Inf Ohm  N_series=1  TIPH1=0 1/K  EG=1.11 eV  TXIS1=3  TXIS2=3  TRS1=0  TRP1=0  Tmeas=25 C  TFIXED=25 C  thermal_mass=100 J/K  initial_temperature=25 degC
      settings: SourceProductName=Simscape Electrical  SourceProductBaseCode=PS
  Conn1 : PMIOPort  Side=Left
  Conn2 : PMIOPort  Port=2  Side=Right
  Conn3 : PMIOPort  Port=3  Side=Left
  connections:
  Solar Cell/LConn2 -- Conn2/RConn1
  Solar Cell/LConn1 -- Conn1/RConn1 -- Solar Cell2/LConn1 -- Solar Cell1/LConn1
  Solar Cell1/RConn1 -- Solar Cell2/LConn2
  Solar Cell/RConn1 -- Solar Cell1/LConn2
  Solar Cell2/RConn1 -- Conn3/RConn1

== system PV_solarpannel/Subsystem3/Subsystem9/Subsystem4 ==
  Solar Cell : ee_lib/Sources/Solar Cell  prm=1  Isc=6 A  Voc=0.6 V  Is=1e-6 A  Is2=0 A  Iph=7.34 A  Ir0=1000 W/m^2  ec=1.5  N2=2  Rs=0 Ohm  Rp=Inf Ohm  N_series=1  TIPH1=0 1/K  EG=1.11 eV  TXIS1=3  TXIS2=3  TRS1=0  TRP1=0  Tmeas=25 C  TFIXED=25 C  thermal_mass=100 J/K  initial_temperature=25 degC
      settings: SourceProductName=Simscape Electrical  SourceProductBaseCode=PS
  Solar Cell1 : ee_lib/Sources/Solar Cell  prm=1  Isc=6 A  Voc=0.6 V  Is=1e-6 A  Is2=0 A  Iph=7.34 A  Ir0=1000 W/m^2  ec=1.5  N2=2  Rs=0 Ohm  Rp=Inf Ohm  N_series=1  TIPH1=0 1/K  EG=1.11 eV  TXIS1=3  TXIS2=3  TRS1=0  TRP1=0  Tmeas=25 C  TFIXED=25 C  thermal_mass=100 J/K  initial_temperature=25 degC
      settings: SourceProductName=Simscape Electrical  SourceProductBaseCode=PS
  Solar Cell2 : ee_lib/Sources/Solar Cell  prm=1  Isc=6 A  Voc=0.6 V  Is=1e-6 A  Is2=0 A  Iph=7.34 A  Ir0=1000 W/m^2  ec=1.5  N2=2  Rs=0 Ohm  Rp=Inf Ohm  N_series=1  TIPH1=0 1/K  EG=1.11 eV  TXIS1=3  TXIS2=3  TRS1=0  TRP1=0  Tmeas=25 C  TFIXED=25 C  thermal_mass=100 J/K  initial_temperature=25 degC
      settings: SourceProductName=Simscape Electrical  SourceProductBaseCode=PS
  Conn1 : PMIOPort  Side=Left
  Conn2 : PMIOPort  Port=2  Side=Right
  Conn3 : PMIOPort  Port=3  Side=Left
  connections:
  Solar Cell/LConn2 -- Conn2/RConn1
  Solar Cell/LConn1 -- Conn1/RConn1 -- Solar Cell2/LConn1 -- Solar Cell1/LConn1
  Solar Cell1/RConn1 -- Solar Cell2/LConn2
  Solar Cell/RConn1 -- Solar Cell1/LConn2
  Solar Cell2/RConn1 -- Conn3/RConn1

== system PV_solarpannel/Subsystem3/Subsystem9/Subsystem5 ==
  Solar Cell : ee_lib/Sources/Solar Cell  prm=1  Isc=6 A  Voc=0.6 V  Is=1e-6 A  Is2=0 A  Iph=7.34 A  Ir0=1000 W/m^2  ec=1.5  N2=2  Rs=0 Ohm  Rp=Inf Ohm  N_series=1  TIPH1=0 1/K  EG=1.11 eV  TXIS1=3  TXIS2=3  TRS1=0  TRP1=0  Tmeas=25 C  TFIXED=25 C  thermal_mass=100 J/K  initial_temperature=25 degC
      settings: SourceProductName=Simscape Electrical  SourceProductBaseCode=PS
  Solar Cell1 : ee_lib/Sources/Solar Cell  prm=1  Isc=6 A  Voc=0.6 V  Is=1e-6 A  Is2=0 A  Iph=7.34 A  Ir0=1000 W/m^2  ec=1.5  N2=2  Rs=0 Ohm  Rp=Inf Ohm  N_series=1  TIPH1=0 1/K  EG=1.11 eV  TXIS1=3  TXIS2=3  TRS1=0  TRP1=0  Tmeas=25 C  TFIXED=25 C  thermal_mass=100 J/K  initial_temperature=25 degC
      settings: SourceProductName=Simscape Electrical  SourceProductBaseCode=PS
  Solar Cell2 : ee_lib/Sources/Solar Cell  prm=1  Isc=6 A  Voc=0.6 V  Is=1e-6 A  Is2=0 A  Iph=7.34 A  Ir0=1000 W/m^2  ec=1.5  N2=2  Rs=0 Ohm  Rp=Inf Ohm  N_series=1  TIPH1=0 1/K  EG=1.11 eV  TXIS1=3  TXIS2=3  TRS1=0  TRP1=0  Tmeas=25 C  TFIXED=25 C  thermal_mass=100 J/K  initial_temperature=25 degC
      settings: SourceProductName=Simscape Electrical  SourceProductBaseCode=PS
  Conn1 : PMIOPort  Side=Left
  Conn2 : PMIOPort  Port=2  Side=Right
  Conn3 : PMIOPort  Port=3  Side=Left
  connections:
  Solar Cell/LConn2 -- Conn2/RConn1
  Solar Cell/LConn1 -- Conn1/RConn1 -- Solar Cell2/LConn1 -- Solar Cell1/LConn1
  Solar Cell1/RConn1 -- Solar Cell2/LConn2
  Solar Cell/RConn1 -- Solar Cell1/LConn2
  Solar Cell2/RConn1 -- Conn3/RConn1

== system PV_solarpannel/Subsystem3/Subsystem9/Subsystem6 ==
  Solar Cell : ee_lib/Sources/Solar Cell  prm=1  Isc=6 A  Voc=0.6 V  Is=1e-6 A  Is2=0 A  Iph=7.34 A  Ir0=1000 W/m^2  ec=1.5  N2=2  Rs=0 Ohm  Rp=Inf Ohm  N_series=1  TIPH1=0 1/K  EG=1.11 eV  TXIS1=3  TXIS2=3  TRS1=0  TRP1=0  Tmeas=25 C  TFIXED=25 C  thermal_mass=100 J/K  initial_temperature=25 degC
      settings: SourceProductName=Simscape Electrical  SourceProductBaseCode=PS
  Solar Cell1 : ee_lib/Sources/Solar Cell  prm=1  Isc=6 A  Voc=0.6 V  Is=1e-6 A  Is2=0 A  Iph=7.34 A  Ir0=1000 W/m^2  ec=1.5  N2=2  Rs=0 Ohm  Rp=Inf Ohm  N_series=1  TIPH1=0 1/K  EG=1.11 eV  TXIS1=3  TXIS2=3  TRS1=0  TRP1=0  Tmeas=25 C  TFIXED=25 C  thermal_mass=100 J/K  initial_temperature=25 degC
      settings: SourceProductName=Simscape Electrical  SourceProductBaseCode=PS
  Solar Cell2 : ee_lib/Sources/Solar Cell  prm=1  Isc=6 A  Voc=0.6 V  Is=1e-6 A  Is2=0 A  Iph=7.34 A  Ir0=1000 W/m^2  ec=1.5  N2=2  Rs=0 Ohm  Rp=Inf Ohm  N_series=1  TIPH1=0 1/K  EG=1.11 eV  TXIS1=3  TXIS2=3  TRS1=0  TRP1=0  Tmeas=25 C  TFIXED=25 C  thermal_mass=100 J/K  initial_temperature=25 degC
      settings: SourceProductName=Simscape Electrical  SourceProductBaseCode=PS
  Conn1 : PMIOPort  Side=Left
  Conn2 : PMIOPort  Port=2  Side=Right
  Conn3 : PMIOPort  Port=3  Side=Left
  connections:
  Solar Cell/LConn2 -- Conn2/RConn1
  Solar Cell/LConn1 -- Conn1/RConn1 -- Solar Cell2/LConn1 -- Solar Cell1/LConn1
  Solar Cell1/RConn1 -- Solar Cell2/LConn2
  Solar Cell/RConn1 -- Solar Cell1/LConn2
  Solar Cell2/RConn1 -- Conn3/RConn1

== system PV_solarpannel/Subsystem3/Subsystem9/Subsystem7 ==
  Solar Cell : ee_lib/Sources/Solar Cell  prm=1  Isc=6 A  Voc=0.6 V  Is=1e-6 A  Is2=0 A  Iph=7.34 A  Ir0=1000 W/m^2  ec=1.5  N2=2  Rs=0 Ohm  Rp=Inf Ohm  N_series=1  TIPH1=0 1/K  EG=1.11 eV  TXIS1=3  TXIS2=3  TRS1=0  TRP1=0  Tmeas=25 C  TFIXED=25 C  thermal_mass=100 J/K  initial_temperature=25 degC
      settings: SourceProductName=Simscape Electrical  SourceProductBaseCode=PS
  Solar Cell1 : ee_lib/Sources/Solar Cell  prm=1  Isc=6 A  Voc=0.6 V  Is=1e-6 A  Is2=0 A  Iph=7.34 A  Ir0=1000 W/m^2  ec=1.5  N2=2  Rs=0 Ohm  Rp=Inf Ohm  N_series=1  TIPH1=0 1/K  EG=1.11 eV  TXIS1=3  TXIS2=3  TRS1=0  TRP1=0  Tmeas=25 C  TFIXED=25 C  thermal_mass=100 J/K  initial_temperature=25 degC
      settings: SourceProductName=Simscape Electrical  SourceProductBaseCode=PS
  Solar Cell2 : ee_lib/Sources/Solar Cell  prm=1  Isc=6 A  Voc=0.6 V  Is=1e-6 A  Is2=0 A  Iph=7.34 A  Ir0=1000 W/m^2  ec=1.5  N2=2  Rs=0 Ohm  Rp=Inf Ohm  N_series=1  TIPH1=0 1/K  EG=1.11 eV  TXIS1=3  TXIS2=3  TRS1=0  TRP1=0  Tmeas=25 C  TFIXED=25 C  thermal_mass=100 J/K  initial_temperature=25 degC
      settings: SourceProductName=Simscape Electrical  SourceProductBaseCode=PS
  Conn1 : PMIOPort  Side=Left
  Conn2 : PMIOPort  Port=2  Side=Right
  Conn3 : PMIOPort  Port=3  Side=Left
  connections:
  Solar Cell/LConn2 -- Conn2/RConn1
  Solar Cell/LConn1 -- Conn1/RConn1 -- Solar Cell2/LConn1 -- Solar Cell1/LConn1
  Solar Cell1/RConn1 -- Solar Cell2/LConn2
  Solar Cell/RConn1 -- Solar Cell1/LConn2
  Solar Cell2/RConn1 -- Conn3/RConn1

== system PV_solarpannel/Subsystem3/Subsystem9/Subsystem8 ==
  Solar Cell : ee_lib/Sources/Solar Cell  prm=1  Isc=6 A  Voc=0.6 V  Is=1e-6 A  Is2=0 A  Iph=7.34 A  Ir0=1000 W/m^2  ec=1.5  N2=2  Rs=0 Ohm  Rp=Inf Ohm  N_series=1  TIPH1=0 1/K  EG=1.11 eV  TXIS1=3  TXIS2=3  TRS1=0  TRP1=0  Tmeas=25 C  TFIXED=25 C  thermal_mass=100 J/K  initial_temperature=25 degC
      settings: SourceProductName=Simscape Electrical  SourceProductBaseCode=PS
  Solar Cell1 : ee_lib/Sources/Solar Cell  prm=1  Isc=6 A  Voc=0.6 V  Is=1e-6 A  Is2=0 A  Iph=7.34 A  Ir0=1000 W/m^2  ec=1.5  N2=2  Rs=0 Ohm  Rp=Inf Ohm  N_series=1  TIPH1=0 1/K  EG=1.11 eV  TXIS1=3  TXIS2=3  TRS1=0  TRP1=0  Tmeas=25 C  TFIXED=25 C  thermal_mass=100 J/K  initial_temperature=25 degC
      settings: SourceProductName=Simscape Electrical  SourceProductBaseCode=PS
  Solar Cell2 : ee_lib/Sources/Solar Cell  prm=1  Isc=6 A  Voc=0.6 V  Is=1e-6 A  Is2=0 A  Iph=7.34 A  Ir0=1000 W/m^2  ec=1.5  N2=2  Rs=0 Ohm  Rp=Inf Ohm  N_series=1  TIPH1=0 1/K  EG=1.11 eV  TXIS1=3  TXIS2=3  TRS1=0  TRP1=0  Tmeas=25 C  TFIXED=25 C  thermal_mass=100 J/K  initial_temperature=25 degC
      settings: SourceProductName=Simscape Electrical  SourceProductBaseCode=PS
  Conn1 : PMIOPort  Side=Left
  Conn2 : PMIOPort  Port=2  Side=Right
  Conn3 : PMIOPort  Port=3  Side=Left
  connections:
  Solar Cell/LConn2 -- Conn2/RConn1
  Solar Cell/LConn1 -- Conn1/RConn1 -- Solar Cell2/LConn1 -- Solar Cell1/LConn1
  Solar Cell1/RConn1 -- Solar Cell2/LConn2
  Solar Cell/RConn1 -- Solar Cell1/LConn2
  Solar Cell2/RConn1 -- Conn3/RConn1

== system PV_solarpannel/Subsystem4/Subsystem9/Subsystem ==
  Solar Cell : ee_lib/Sources/Solar Cell  prm=1  Isc=6 A  Voc=0.6 V  Is=1e-6 A  Is2=0 A  Iph=7.34 A  Ir0=1000 W/m^2  ec=1.5  N2=2  Rs=0 Ohm  Rp=Inf Ohm  N_series=1  TIPH1=0 1/K  EG=1.11 eV  TXIS1=3  TXIS2=3  TRS1=0  TRP1=0  Tmeas=25 C  TFIXED=25 C  thermal_mass=100 J/K  initial_temperature=25 degC
      settings: SourceProductName=Simscape Electrical  SourceProductBaseCode=PS
  Solar Cell1 : ee_lib/Sources/Solar Cell  prm=1  Isc=6 A  Voc=0.6 V  Is=1e-6 A  Is2=0 A  Iph=7.34 A  Ir0=1000 W/m^2  ec=1.5  N2=2  Rs=0 Ohm  Rp=Inf Ohm  N_series=1  TIPH1=0 1/K  EG=1.11 eV  TXIS1=3  TXIS2=3  TRS1=0  TRP1=0  Tmeas=25 C  TFIXED=25 C  thermal_mass=100 J/K  initial_temperature=25 degC
      settings: SourceProductName=Simscape Electrical  SourceProductBaseCode=PS
  Solar Cell2 : ee_lib/Sources/Solar Cell  prm=1  Isc=6 A  Voc=0.6 V  Is=1e-6 A  Is2=0 A  Iph=7.34 A  Ir0=1000 W/m^2  ec=1.5  N2=2  Rs=0 Ohm  Rp=Inf Ohm  N_series=1  TIPH1=0 1/K  EG=1.11 eV  TXIS1=3  TXIS2=3  TRS1=0  TRP1=0  Tmeas=25 C  TFIXED=25 C  thermal_mass=100 J/K  initial_temperature=25 degC
      settings: SourceProductName=Simscape Electrical  SourceProductBaseCode=PS
  Conn1 : PMIOPort  Side=Left
  Conn2 : PMIOPort  Port=2  Side=Right
  Conn3 : PMIOPort  Port=3  Side=Left
  connections:
  Solar Cell/LConn2 -- Conn2/RConn1
  Solar Cell/LConn1 -- Conn1/RConn1 -- Solar Cell2/LConn1 -- Solar Cell1/LConn1
  Solar Cell1/RConn1 -- Solar Cell2/LConn2
  Solar Cell/RConn1 -- Solar Cell1/LConn2
  Solar Cell2/RConn1 -- Conn3/RConn1

== system PV_solarpannel/Subsystem4/Subsystem9/Subsystem1 ==
  Solar Cell : ee_lib/Sources/Solar Cell  prm=1  Isc=6 A  Voc=0.6 V  Is=1e-6 A  Is2=0 A  Iph=7.34 A  Ir0=1000 W/m^2  ec=1.5  N2=2  Rs=0 Ohm  Rp=Inf Ohm  N_series=1  TIPH1=0 1/K  EG=1.11 eV  TXIS1=3  TXIS2=3  TRS1=0  TRP1=0  Tmeas=25 C  TFIXED=25 C  thermal_mass=100 J/K  initial_temperature=25 degC
      settings: SourceProductName=Simscape Electrical  SourceProductBaseCode=PS
  Solar Cell1 : ee_lib/Sources/Solar Cell  prm=1  Isc=6 A  Voc=0.6 V  Is=1e-6 A  Is2=0 A  Iph=7.34 A  Ir0=1000 W/m^2  ec=1.5  N2=2  Rs=0 Ohm  Rp=Inf Ohm  N_series=1  TIPH1=0 1/K  EG=1.11 eV  TXIS1=3  TXIS2=3  TRS1=0  TRP1=0  Tmeas=25 C  TFIXED=25 C  thermal_mass=100 J/K  initial_temperature=25 degC
      settings: SourceProductName=Simscape Electrical  SourceProductBaseCode=PS
  Solar Cell2 : ee_lib/Sources/Solar Cell  prm=1  Isc=6 A  Voc=0.6 V  Is=1e-6 A  Is2=0 A  Iph=7.34 A  Ir0=1000 W/m^2  ec=1.5  N2=2  Rs=0 Ohm  Rp=Inf Ohm  N_series=1  TIPH1=0 1/K  EG=1.11 eV  TXIS1=3  TXIS2=3  TRS1=0  TRP1=0  Tmeas=25 C  TFIXED=25 C  thermal_mass=100 J/K  initial_temperature=25 degC
      settings: SourceProductName=Simscape Electrical  SourceProductBaseCode=PS
  Conn1 : PMIOPort  Side=Left
  Conn2 : PMIOPort  Port=2  Side=Right
  Conn3 : PMIOPort  Port=3  Side=Left
  connections:
  Solar Cell2/RConn1 -- Conn3/RConn1
  Solar Cell/RConn1 -- Solar Cell1/LConn2
  Solar Cell1/RConn1 -- Solar Cell2/LConn2
  Conn1/RConn1 -- Solar Cell/LConn1 -- Solar Cell1/LConn1 -- Solar Cell2/LConn1
  Solar Cell/LConn2 -- Conn2/RConn1

== system PV_solarpannel/Subsystem4/Subsystem9/Subsystem2 ==
  Solar Cell : ee_lib/Sources/Solar Cell  prm=1  Isc=6 A  Voc=0.6 V  Is=1e-6 A  Is2=0 A  Iph=7.34 A  Ir0=1000 W/m^2  ec=1.5  N2=2  Rs=0 Ohm  Rp=Inf Ohm  N_series=1  TIPH1=0 1/K  EG=1.11 eV  TXIS1=3  TXIS2=3  TRS1=0  TRP1=0  Tmeas=25 C  TFIXED=25 C  thermal_mass=100 J/K  initial_temperature=25 degC
      settings: SourceProductName=Simscape Electrical  SourceProductBaseCode=PS
  Solar Cell1 : ee_lib/Sources/Solar Cell  prm=1  Isc=6 A  Voc=0.6 V  Is=1e-6 A  Is2=0 A  Iph=7.34 A  Ir0=1000 W/m^2  ec=1.5  N2=2  Rs=0 Ohm  Rp=Inf Ohm  N_series=1  TIPH1=0 1/K  EG=1.11 eV  TXIS1=3  TXIS2=3  TRS1=0  TRP1=0  Tmeas=25 C  TFIXED=25 C  thermal_mass=100 J/K  initial_temperature=25 degC
      settings: SourceProductName=Simscape Electrical  SourceProductBaseCode=PS
  Solar Cell2 : ee_lib/Sources/Solar Cell  prm=1  Isc=6 A  Voc=0.6 V  Is=1e-6 A  Is2=0 A  Iph=7.34 A  Ir0=1000 W/m^2  ec=1.5  N2=2  Rs=0 Ohm  Rp=Inf Ohm  N_series=1  TIPH1=0 1/K  EG=1.11 eV  TXIS1=3  TXIS2=3  TRS1=0  TRP1=0  Tmeas=25 C  TFIXED=25 C  thermal_mass=100 J/K  initial_temperature=25 degC
      settings: SourceProductName=Simscape Electrical  SourceProductBaseCode=PS
  Conn1 : PMIOPort  Side=Left
  Conn2 : PMIOPort  Port=2  Side=Right
  Conn3 : PMIOPort  Port=3  Side=Left
  connections:
  Solar Cell/LConn2 -- Conn2/RConn1
  Solar Cell2/LConn1 -- Solar Cell1/LConn1 -- Solar Cell/LConn1 -- Conn1/RConn1
  Solar Cell1/RConn1 -- Solar Cell2/LConn2
  Solar Cell/RConn1 -- Solar Cell1/LConn2
  Solar Cell2/RConn1 -- Conn3/RConn1

== system PV_solarpannel/Subsystem4/Subsystem9/Subsystem3 ==
  Solar Cell : ee_lib/Sources/Solar Cell  prm=1  Isc=6 A  Voc=0.6 V  Is=1e-6 A  Is2=0 A  Iph=7.34 A  Ir0=1000 W/m^2  ec=1.5  N2=2  Rs=0 Ohm  Rp=Inf Ohm  N_series=1  TIPH1=0 1/K  EG=1.11 eV  TXIS1=3  TXIS2=3  TRS1=0  TRP1=0  Tmeas=25 C  TFIXED=25 C  thermal_mass=100 J/K  initial_temperature=25 degC
      settings: SourceProductName=Simscape Electrical  SourceProductBaseCode=PS
  Solar Cell1 : ee_lib/Sources/Solar Cell  prm=1  Isc=6 A  Voc=0.6 V  Is=1e-6 A  Is2=0 A  Iph=7.34 A  Ir0=1000 W/m^2  ec=1.5  N2=2  Rs=0 Ohm  Rp=Inf Ohm  N_series=1  TIPH1=0 1/K  EG=1.11 eV  TXIS1=3  TXIS2=3  TRS1=0  TRP1=0  Tmeas=25 C  TFIXED=25 C  thermal_mass=100 J/K  initial_temperature=25 degC
      settings: SourceProductName=Simscape Electrical  SourceProductBaseCode=PS
  Solar Cell2 : ee_lib/Sources/Solar Cell  prm=1  Isc=6 A  Voc=0.6 V  Is=1e-6 A  Is2=0 A  Iph=7.34 A  Ir0=1000 W/m^2  ec=1.5  N2=2  Rs=0 Ohm  Rp=Inf Ohm  N_series=1  TIPH1=0 1/K  EG=1.11 eV  TXIS1=3  TXIS2=3  TRS1=0  TRP1=0  Tmeas=25 C  TFIXED=25 C  thermal_mass=100 J/K  initial_temperature=25 degC
      settings: SourceProductName=Simscape Electrical  SourceProductBaseCode=PS
  Conn1 : PMIOPort  Side=Left
  Conn2 : PMIOPort  Port=2  Side=Right
  Conn3 : PMIOPort  Port=3  Side=Left
  connections:
  Solar Cell/LConn2 -- Conn2/RConn1
  Solar Cell/LConn1 -- Conn1/RConn1 -- Solar Cell2/LConn1 -- Solar Cell1/LConn1
  Solar Cell1/RConn1 -- Solar Cell2/LConn2
  Solar Cell/RConn1 -- Solar Cell1/LConn2
  Solar Cell2/RConn1 -- Conn3/RConn1

== system PV_solarpannel/Subsystem4/Subsystem9/Subsystem4 ==
  Solar Cell : ee_lib/Sources/Solar Cell  prm=1  Isc=6 A  Voc=0.6 V  Is=1e-6 A  Is2=0 A  Iph=7.34 A  Ir0=1000 W/m^2  ec=1.5  N2=2  Rs=0 Ohm  Rp=Inf Ohm  N_series=1  TIPH1=0 1/K  EG=1.11 eV  TXIS1=3  TXIS2=3  TRS1=0  TRP1=0  Tmeas=25 C  TFIXED=25 C  thermal_mass=100 J/K  initial_temperature=25 degC
      settings: SourceProductName=Simscape Electrical  SourceProductBaseCode=PS
  Solar Cell1 : ee_lib/Sources/Solar Cell  prm=1  Isc=6 A  Voc=0.6 V  Is=1e-6 A  Is2=0 A  Iph=7.34 A  Ir0=1000 W/m^2  ec=1.5  N2=2  Rs=0 Ohm  Rp=Inf Ohm  N_series=1  TIPH1=0 1/K  EG=1.11 eV  TXIS1=3  TXIS2=3  TRS1=0  TRP1=0  Tmeas=25 C  TFIXED=25 C  thermal_mass=100 J/K  initial_temperature=25 degC
      settings: SourceProductName=Simscape Electrical  SourceProductBaseCode=PS
  Solar Cell2 : ee_lib/Sources/Solar Cell  prm=1  Isc=6 A  Voc=0.6 V  Is=1e-6 A  Is2=0 A  Iph=7.34 A  Ir0=1000 W/m^2  ec=1.5  N2=2  Rs=0 Ohm  Rp=Inf Ohm  N_series=1  TIPH1=0 1/K  EG=1.11 eV  TXIS1=3  TXIS2=3  TRS1=0  TRP1=0  Tmeas=25 C  TFIXED=25 C  thermal_mass=100 J/K  initial_temperature=25 degC
      settings: SourceProductName=Simscape Electrical  SourceProductBaseCode=PS
  Conn1 : PMIOPort  Side=Left
  Conn2 : PMIOPort  Port=2  Side=Right
  Conn3 : PMIOPort  Port=3  Side=Left
  connections:
  Solar Cell/LConn2 -- Conn2/RConn1
  Solar Cell/LConn1 -- Conn1/RConn1 -- Solar Cell2/LConn1 -- Solar Cell1/LConn1
  Solar Cell1/RConn1 -- Solar Cell2/LConn2
  Solar Cell/RConn1 -- Solar Cell1/LConn2
  Solar Cell2/RConn1 -- Conn3/RConn1

== system PV_solarpannel/Subsystem4/Subsystem9/Subsystem5 ==
  Solar Cell : ee_lib/Sources/Solar Cell  prm=1  Isc=6 A  Voc=0.6 V  Is=1e-6 A  Is2=0 A  Iph=7.34 A  Ir0=1000 W/m^2  ec=1.5  N2=2  Rs=0 Ohm  Rp=Inf Ohm  N_series=1  TIPH1=0 1/K  EG=1.11 eV  TXIS1=3  TXIS2=3  TRS1=0  TRP1=0  Tmeas=25 C  TFIXED=25 C  thermal_mass=100 J/K  initial_temperature=25 degC
      settings: SourceProductName=Simscape Electrical  SourceProductBaseCode=PS
  Solar Cell1 : ee_lib/Sources/Solar Cell  prm=1  Isc=6 A  Voc=0.6 V  Is=1e-6 A  Is2=0 A  Iph=7.34 A  Ir0=1000 W/m^2  ec=1.5  N2=2  Rs=0 Ohm  Rp=Inf Ohm  N_series=1  TIPH1=0 1/K  EG=1.11 eV  TXIS1=3  TXIS2=3  TRS1=0  TRP1=0  Tmeas=25 C  TFIXED=25 C  thermal_mass=100 J/K  initial_temperature=25 degC
      settings: SourceProductName=Simscape Electrical  SourceProductBaseCode=PS
  Solar Cell2 : ee_lib/Sources/Solar Cell  prm=1  Isc=6 A  Voc=0.6 V  Is=1e-6 A  Is2=0 A  Iph=7.34 A  Ir0=1000 W/m^2  ec=1.5  N2=2  Rs=0 Ohm  Rp=Inf Ohm  N_series=1  TIPH1=0 1/K  EG=1.11 eV  TXIS1=3  TXIS2=3  TRS1=0  TRP1=0  Tmeas=25 C  TFIXED=25 C  thermal_mass=100 J/K  initial_temperature=25 degC
      settings: SourceProductName=Simscape Electrical  SourceProductBaseCode=PS
  Conn1 : PMIOPort  Side=Left
  Conn2 : PMIOPort  Port=2  Side=Right
  Conn3 : PMIOPort  Port=3  Side=Left
  connections:
  Solar Cell/LConn2 -- Conn2/RConn1
  Solar Cell/LConn1 -- Conn1/RConn1 -- Solar Cell2/LConn1 -- Solar Cell1/LConn1
  Solar Cell1/RConn1 -- Solar Cell2/LConn2
  Solar Cell/RConn1 -- Solar Cell1/LConn2
  Solar Cell2/RConn1 -- Conn3/RConn1

== system PV_solarpannel/Subsystem4/Subsystem9/Subsystem6 ==
  Solar Cell : ee_lib/Sources/Solar Cell  prm=1  Isc=6 A  Voc=0.6 V  Is=1e-6 A  Is2=0 A  Iph=7.34 A  Ir0=1000 W/m^2  ec=1.5  N2=2  Rs=0 Ohm  Rp=Inf Ohm  N_series=1  TIPH1=0 1/K  EG=1.11 eV  TXIS1=3  TXIS2=3  TRS1=0  TRP1=0  Tmeas=25 C  TFIXED=25 C  thermal_mass=100 J/K  initial_temperature=25 degC
      settings: SourceProductName=Simscape Electrical  SourceProductBaseCode=PS
  Solar Cell1 : ee_lib/Sources/Solar Cell  prm=1  Isc=6 A  Voc=0.6 V  Is=1e-6 A  Is2=0 A  Iph=7.34 A  Ir0=1000 W/m^2  ec=1.5  N2=2  Rs=0 Ohm  Rp=Inf Ohm  N_series=1  TIPH1=0 1/K  EG=1.11 eV  TXIS1=3  TXIS2=3  TRS1=0  TRP1=0  Tmeas=25 C  TFIXED=25 C  thermal_mass=100 J/K  initial_temperature=25 degC
      settings: SourceProductName=Simscape Electrical  SourceProductBaseCode=PS
  Solar Cell2 : ee_lib/Sources/Solar Cell  prm=1  Isc=6 A  Voc=0.6 V  Is=1e-6 A  Is2=0 A  Iph=7.34 A  Ir0=1000 W/m^2  ec=1.5  N2=2  Rs=0 Ohm  Rp=Inf Ohm  N_series=1  TIPH1=0 1/K  EG=1.11 eV  TXIS1=3  TXIS2=3  TRS1=0  TRP1=0  Tmeas=25 C  TFIXED=25 C  thermal_mass=100 J/K  initial_temperature=25 degC
      settings: SourceProductName=Simscape Electrical  SourceProductBaseCode=PS
  Conn1 : PMIOPort  Side=Left
  Conn2 : PMIOPort  Port=2  Side=Right
  Conn3 : PMIOPort  Port=3  Side=Left
  connections:
  Solar Cell/LConn2 -- Conn2/RConn1
  Solar Cell/LConn1 -- Conn1/RConn1 -- Solar Cell2/LConn1 -- Solar Cell1/LConn1
  Solar Cell1/RConn1 -- Solar Cell2/LConn2
  Solar Cell/RConn1 -- Solar Cell1/LConn2
  Solar Cell2/RConn1 -- Conn3/RConn1

== system PV_solarpannel/Subsystem4/Subsystem9/Subsystem7 ==
  Solar Cell : ee_lib/Sources/Solar Cell  prm=1  Isc=6 A  Voc=0.6 V  Is=1e-6 A  Is2=0 A  Iph=7.34 A  Ir0=1000 W/m^2  ec=1.5  N2=2  Rs=0 Ohm  Rp=Inf Ohm  N_series=1  TIPH1=0 1/K  EG=1.11 eV  TXIS1=3  TXIS2=3  TRS1=0  TRP1=0  Tmeas=25 C  TFIXED=25 C  thermal_mass=100 J/K  initial_temperature=25 degC
      settings: SourceProductName=Simscape Electrical  SourceProductBaseCode=PS
  Solar Cell1 : ee_lib/Sources/Solar Cell  prm=1  Isc=6 A  Voc=0.6 V  Is=1e-6 A  Is2=0 A  Iph=7.34 A  Ir0=1000 W/m^2  ec=1.5  N2=2  Rs=0 Ohm  Rp=Inf Ohm  N_series=1  TIPH1=0 1/K  EG=1.11 eV  TXIS1=3  TXIS2=3  TRS1=0  TRP1=0  Tmeas=25 C  TFIXED=25 C  thermal_mass=100 J/K  initial_temperature=25 degC
      settings: SourceProductName=Simscape Electrical  SourceProductBaseCode=PS
  Solar Cell2 : ee_lib/Sources/Solar Cell  prm=1  Isc=6 A  Voc=0.6 V  Is=1e-6 A  Is2=0 A  Iph=7.34 A  Ir0=1000 W/m^2  ec=1.5  N2=2  Rs=0 Ohm  Rp=Inf Ohm  N_series=1  TIPH1=0 1/K  EG=1.11 eV  TXIS1=3  TXIS2=3  TRS1=0  TRP1=0  Tmeas=25 C  TFIXED=25 C  thermal_mass=100 J/K  initial_temperature=25 degC
      settings: SourceProductName=Simscape Electrical  SourceProductBaseCode=PS
  Conn1 : PMIOPort  Side=Left
  Conn2 : PMIOPort  Port=2  Side=Right
  Conn3 : PMIOPort  Port=3  Side=Left
  connections:
  Solar Cell/LConn2 -- Conn2/RConn1
  Solar Cell/LConn1 -- Conn1/RConn1 -- Solar Cell2/LConn1 -- Solar Cell1/LConn1
  Solar Cell1/RConn1 -- Solar Cell2/LConn2
  Solar Cell/RConn1 -- Solar Cell1/LConn2
  Solar Cell2/RConn1 -- Conn3/RConn1
